simulink model "fuel_cell_vehicle"  (R2024a)
settings: Solver=VariableStepAuto  StartTime=0.0  StopTime=2474  RelTol=1e-3
libraries: autolibshared x1, slpidlib x1
settings Model: Creator=lenovo  LastModifiedBy=lenovo

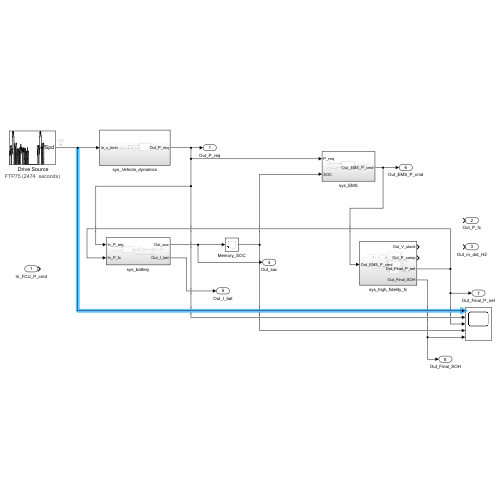
[thumbnail: Simulink's stored preview of the top-level diagram]
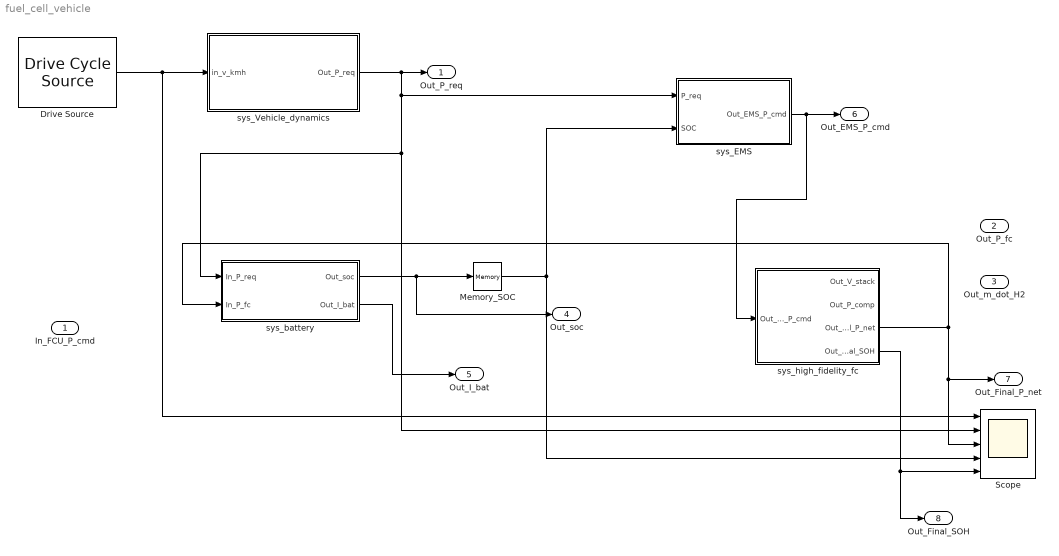
== system fuel_cell_vehicle ==
  In_FCU_P_cmd : Inport
  " Drive Source" : autolibshared/Drive Cycle Source  cycleVar=FTP75  fileVar=cycleFTP75.mat  tfinal="2474  seconds"  cycleRepeat=off  outAccPort=off  outGearPort=off  gearList=No gear data  t_wot1=5  xdot_woto=0  xdot_wot1=30  t_wot2=20  xdot_wot2=0  t_wotend=30  srcUnit=m/s  outUnit=m/s  srcAccUnit=m/s/s  outAccUnit=m/s^2  dt=0  aMode=1  faultOption=off  velBnd=2  velBndUnit=mph  inUnit=m/s  timeBnd=1  failOption=off  stopSim=off  maxFaultCnt=10  maxFaultTime=2  maxTotFaultTime=15  traceOption=off  dtTrace=1  traceWindow=10  lastDCname=FTP75  lastOutUnit=mph  lastDT=0  lastTB=1  lastSB=2  forceCalcBound=off
  Memory_SOC : Memory
  Scope : Scope  NumInputPorts=5
  sys_EMS : Subsystem
  sys_Vehicle_dynamics : Subsystem
  sys_battery : Subsystem
  sys_high_fidelity_fc : Subsystem
  Out_P_req : Outport
  Out_P_fc : Outport  Port=2
  Out_m_dot_H2 : Outport  Port=3
  Out_soc : Outport  Port=4
  Out_I_bat : Outport  Port=5
  Out_EMS_P_cmd : Outport  Port=6
  Out_Final_P_net : Outport  Port=7
  Out_Final_SOH : Outport  Port=8
  wires:
  sys_Vehicle_dynamics/1(Out_P_req) -> Scope/2, sys_battery/1(In_P_req), sys_EMS/1(P_req), Out_P_req/1
  sys_high_fidelity_fc/3(Out_Final_P_net) -> sys_battery/2(In_P_fc), Scope/3, Out_Final_P_net/1
  sys_battery/1(Out_soc) -> Memory_SOC/1, Out_soc/1
  sys_battery/2(Out_I_bat) -> Out_I_bat/1
  sys_EMS/1(Out_EMS_P_cmd) -> sys_high_fidelity_fc/1(Out_EMS_P_cmd), Out_EMS_P_cmd/1
  " Drive Source"/1 -> Scope/1, sys_Vehicle_dynamics/1(in_v_kmh)
  Memory_SOC/1 -> Scope/4, sys_EMS/2(SOC)
  sys_high_fidelity_fc/4(Out_Final_SOH) -> Out_Final_SOH/1, Scope/5

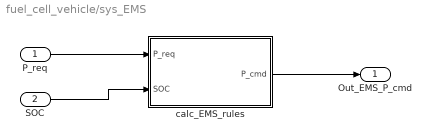
== system fuel_cell_vehicle/sys_EMS ==
  P_req : Inport
  SOC : Inport  Port=2
  calc_EMS_rules : MATLAB Function  TreatAsAtomicUnit=on
  Out_EMS_P_cmd : Outport
  wires:
  calc_EMS_rules/1(P_cmd) -> Out_EMS_P_cmd/1
  P_req/1 -> calc_EMS_rules/1(P_req)
  SOC/1 -> calc_EMS_rules/2(SOC)

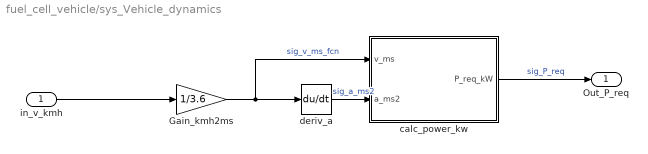
== system fuel_cell_vehicle/sys_Vehicle_dynamics ==
  in_v_kmh : Inport
  Gain_kmh2ms : Gain  Gain=1/3.6
  calc_power_kw : MATLAB Function  TreatAsAtomicUnit=on
  deriv_a : Derivative
  Out_P_req : Outport
  wires:
  in_v_kmh/1 -> Gain_kmh2ms/1
  deriv_a/1 -> calc_power_kw/2(a_ms2)  "sig_a_ms2"
  Gain_kmh2ms/1 -> deriv_a/1, calc_power_kw/1(v_ms)  "sig_v_ms_fcn"
  calc_power_kw/1(P_req_kW) -> Out_P_req/1  "sig_P_req"

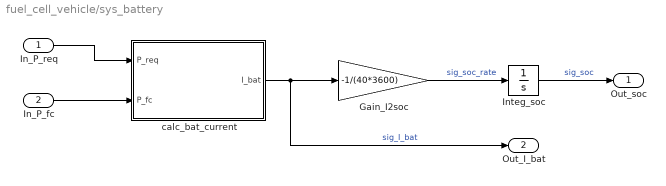
== system fuel_cell_vehicle/sys_battery ==
  In_P_req : Inport
  In_P_fc : Inport  Port=2
  Gain_I2soc : Gain  Gain=-1/(40*3600)
  Integ_soc : Integrator  InitialCondition=0.6
  calc_bat_current : MATLAB Function  TreatAsAtomicUnit=on
  Out_soc : Outport
  Out_I_bat : Outport  Port=2
  wires:
  calc_bat_current/1(I_bat) -> Out_I_bat/1, Gain_I2soc/1  "sig_I_bat"
  Gain_I2soc/1 -> Integ_soc/1  "sig_soc_rate"
  In_P_req/1 -> calc_bat_current/1(P_req)
  Integ_soc/1 -> Out_soc/1  "sig_soc"
  In_P_fc/1 -> calc_bat_current/2(P_fc)

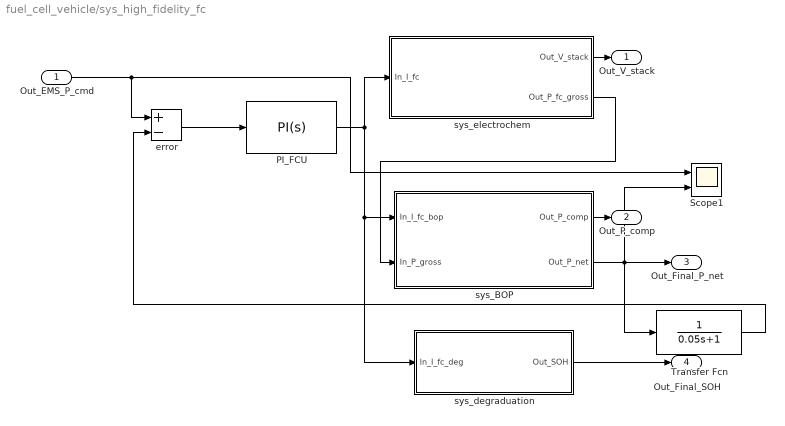
== system fuel_cell_vehicle/sys_high_fidelity_fc ==
  Out_EMS_P_cmd : Inport
  PI_FCU : slpidlib/PID Controller  Controller=PI  Form=Parallel  TimeDomain=Continuous-time  UseExternalTs=off  SampleTime=-1  IntegratorMethod=Forward Euler  FilterMethod=Forward Euler  ControllerParametersSource=internal  P=4  I=3  UseKiTs=off  D=0  UseExternalDerivativeSource=off  N=100  UseFilter=on  TunerSelectOption=Transfer Function Based (PID Tuner App)  InitialConditionSource=internal  InitialConditionForIntegrator=0  InitialConditionForFilter=0  DifferentiatorICPrevScaledInput=0  ExternalReset=none  TrackingMode=off  Kt=1  LimitOutput=on  SatLimitsSource=internal  UpperSaturationLimit=300  LowerSaturationLimit=0  LinearizeAsGain=on  AntiWindupMode=none  Kb=1  LimitIntegrator=off  UpperIntegratorSaturationLimit=inf  LowerIntegratorSaturationLimit=-inf  POutMin=[]  POutMax=[]  IOutMin=[]  IOutMax=[]  DOutMin=[]  DOutMax=[]  NOutMin=[]  NOutMax=[]  SumOutMin=[]  SumOutMax=[]  SaturationOutMin=[]  SaturationOutMax=[]  PParamMin=[]  PParamMax=[]  IParamMin=[]  IParamMax=[]  DParamMin=[]  DParamMax=[]  NParamMin=[]  NParamMax=[]  KbParamMin=[]  KbParamMax=[]  KtParamMin=[]  KtParamMax=[]  KbOutMin=[]  KbOutMax=[]  KtOutMin=[]  KtOutMax=[]  IntegratorOutMin=[]  IntegratorOutMax=[]  FilterOutMin=[]  FilterOutMax=[]  SumI1OutMin=[]  SumI1OutMax=[]  SumI2OutMin=[]  SumI2OutMax=[]  SumI3OutMin=[]  SumI3OutMax=[]  SumI4OutMin=[]  SumI4OutMax=[]  SumDOutMin=[]  SumDOutMax=[]  DifferentiatorOutMin=[]  DifferentiatorOutMax=[]  FilterDiffOutCoefMin=[]  FilterDiffOutCoefMax=[]  ReciprocalOutMin=[]  ReciprocalOutMax=[]  SumDenOutMin=[]  SumDenOutMax=[]  SumNumOutMin=[]  SumNumOutMax=[]  DivideOutMin=[]  DivideOutMax=[]  UdiffTsProdOutMin=[]  UdiffTsProdOutMax=[]  NTsProdOutMin=[]  NTsProdOutMax=[]  UintegralTsProdOutMin=[]  UintegralTsProdOutMax=[]  UngainTsProdOutMin=[]  UngainTsProdOutMax=[]  ClampingZeroOutDataTypeStr=Inherit: Inherit via back propagation  ClampingZeroOutMin=[]  ClampingZeroOutMax=[]  FilterDenConstantOutDataTypeStr=Inherit: Inherit via back propagation  FilterDenConstantOutMin=[]  FilterDenConstantOutMax=[]  PCopyOutDataTypeStr=Inherit: Inherit via back propagation  PCopyOutMin=[]  PCopyOutMax=[]  NCopyOutDataTypeStr=Inherit: Inherit via back propagation  NCopyOutMin=[]  NCopyOutMax=[]  IntegratorContinuousStateAttributes=''  IntegratorStateMustResolveToSignalObject=off  IntegratorRTWStateStorageClass=Auto  FilterContinuousStateAttributes=''  FilterStateMustResolveToSignalObject=off  FilterRTWStateStorageClass=Auto  ParallelPVariant=InternalParameters  IdealPVariant=Disabled  IVariant=InternalParameters  DVariant=Disabled  IntegratorVariant=Continuous  SatVariant=Enabled  AWVariant=Passthrough  PCopyVariant=Disabled  TRVariant=Disabled  FdbkBlocksVariant=Forward  IdealPFdbkVariant=Disabled  SatFdbkVariant=Disabled  DerivativeFilterVariant=Disabled  NVariant=Disabled  NCopyVariant=Disabled_SignalSpec  FilterICVariant=Disabled  IntegratorICVariant=InternalICs  ExternalResetVariant=Disabled  TRSumVariant=Passthrough  SumFdbkVariant=Disabled  SumVariant=Sum_PI  TsampFilterVariant=InternalTs  TsampNgainVariant=Passthrough  TsampIntegralVariant=Disabled_SignalSpec  ExternalSaturationOutDataTypeStr=Inherit: Same as second input  DerivativeSourceVariant=Disabled
  Scope1 : Scope  NumInputPorts=2
  Transfer Fcn : TransferFcn  Denominator=[0.05 1]
  error : Sum  Inputs=+-
  sys_BOP : Subsystem
  sys_degraduation : Subsystem
  sys_electrochem : Subsystem
  Out_V_stack : Outport
  Out_P_comp : Outport  Port=2
  Out_Final_P_net : Outport  Port=3
  Out_Final_SOH : Outport  Port=4
  wires:
  Out_EMS_P_cmd/1 -> Scope1/1, error/1
  PI_FCU/1 -> sys_degraduation/1(In_I_fc_deg), sys_BOP/1(In_I_fc_bop), sys_electrochem/1(In_I_fc)
  error/1 -> PI_FCU/1
  sys_BOP/2(Out_P_net) -> Out_Final_P_net/1, Transfer Fcn/1, Scope1/2
  Transfer Fcn/1 -> error/2
  sys_electrochem/1(Out_V_stack) -> Out_V_stack/1
  sys_electrochem/2(Out_P_fc_gross) -> sys_BOP/2(In_P_gross)
  sys_degraduation/1(Out_SOH) -> Out_Final_SOH/1
  sys_BOP/1(Out_P_comp) -> Out_P_comp/1

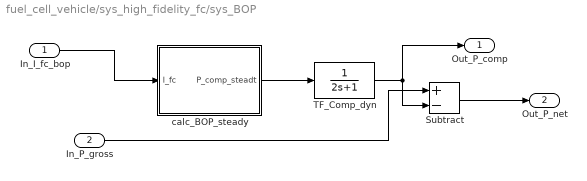
== system fuel_cell_vehicle/sys_high_fidelity_fc/sys_BOP ==
  In_I_fc_bop : Inport
  In_P_gross : Inport  Port=2
  Subtract : Sum  Inputs=+-
  TF_Comp_dyn : TransferFcn  Denominator=[2 1]
  calc_BOP_steady : MATLAB Function  TreatAsAtomicUnit=on
  Out_P_comp : Outport
  Out_P_net : Outport  Port=2
  wires:
  In_P_gross/1 -> Subtract/1
  Subtract/1 -> Out_P_net/1
  calc_BOP_steady/1(P_comp_steadt) -> TF_Comp_dyn/1
  In_I_fc_bop/1 -> calc_BOP_steady/1(I_fc)
  TF_Comp_dyn/1 -> Out_P_comp/1, Subtract/2

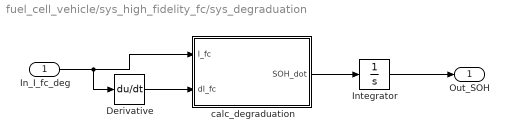
== system fuel_cell_vehicle/sys_high_fidelity_fc/sys_degraduation ==
  In_I_fc_deg : Inport
  Derivative : Derivative
  Integrator : Integrator  InitialCondition=1
  calc_degraduation : MATLAB Function  TreatAsAtomicUnit=on
  Out_SOH : Outport
  wires:
  calc_degraduation/1(SOH_dot) -> Integrator/1
  Integrator/1 -> Out_SOH/1
  In_I_fc_deg/1 -> Derivative/1, calc_degraduation/1(I_fc)
  Derivative/1 -> calc_degraduation/2(dI_fc)

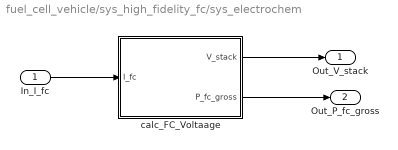
== system fuel_cell_vehicle/sys_high_fidelity_fc/sys_electrochem ==
  In_I_fc : Inport
  calc_FC_Voltaage : MATLAB Function  TreatAsAtomicUnit=on
  Out_V_stack : Outport
  Out_P_fc_gross : Outport  Port=2
  wires:
  calc_FC_Voltaage/2(P_fc_gross) -> Out_P_fc_gross/1
  In_I_fc/1 -> calc_FC_Voltaage/1(I_fc)
  calc_FC_Voltaage/1(V_stack) -> Out_V_stack/1

== matlab function fuel_cell_vehicle/sys_battery/calc_bat_current ==
  data: P_req input; I_bat output; P_fc input
function I_bat = fcn(P_req, P_fc)
    % 电池参数
    U = 300;    % 标称电压 (V)
    R = 0.1;    % 内阻 (Ohm)
    
    % 计算电池实际功率并转换为瓦特 (W)
    P_bat_W = (P_req - P_fc) * 1000;
    
    % 安全保护：防止极端大功率下根号内出现负数导致仿真崩溃
    limit_val = U^2 - 4 * R * P_bat_W;
    if limit_val < 0
        limit_val = 0; 
    end
    
    % 内阻模型计算电流 (A)
    I_bat = (U - sqrt(limit_val)) / (2 * R);
end

== matlab function fuel_cell_vehicle/sys_EMS/calc_EMS_rules ==
  data: P_req input; P_cmd output; SOC input
function P_cmd = fcn(P_req, SOC)
    % EMS 基于规则的控制策略 (Rule-based Control)
    
    % 设定阈值参数
    SOC_low = 0.4;
    SOC_high = 0.8;
    P_fc_max = 50;  % kW
    P_fc_min = 5;   % kW
    P_fc_opt = 25;  % kW
    
    % 状态机控制逻辑
    if SOC < SOC_low
        % 规则1：电量极低，强制全开充电
        P_cmd = P_fc_max;
    elseif SOC > SOC_high
        % 规则2：电量很满
        if P_req > P_fc_max
            % 如果此时车辆猛加速（需求大于FC最大功率），FC全开帮忙，保护电池
            P_cmd = P_fc_max; 
        else
            % 否则FC怠速，纯靠电池放电
            P_cmd = P_fc_min; 
        end
    else
        % 规则3：电量正常 (0.4~0.8区间)
        % 让燃料电池保持在最高效率点，剩余功率波动由电池去扛
        P_cmd = P_fc_opt; 
    end
end

== matlab function fuel_cell_vehicle/sys_high_fidelity_fc/sys_BOP/calc_BOP_steady ==
  data: I_fc input; P_comp_steadt output
function P_comp_steadt = fcn(I_fc)
c0 =0.4;
c1 =0.008;
c2=0.00007;

P_comp_steadt = c0+c1*I_fc+c2*(I_fc^2);

== matlab function fuel_cell_vehicle/sys_high_fidelity_fc/sys_degraduation/calc_degraduation ==
  data: I_fc input; SOH_dot output; dI_fc input
function SOH_dot = fcn(I_fc, dI_fc)
    % 仿真加速因子（放大 10000 倍，以便在短时间仿真中能肉眼看到寿命下降）
    Acc_Factor = 100;
    
    % 寿命衰减参数
    I_opt = 100;         % 最佳健康电流 (A)
    k0 = 5e-7;           % 基础衰减率
    k1 = 2e-11;          % 稳态偏离惩罚系数
    k_trans = 1e-6;      % 动态突变惩罚系数
    
    % 计算稳态衰减 (偏离 100A 越远，衰减越快)
    k_steady = k0 + k1 * (I_fc - I_opt)^2;
    
    % 计算瞬态突变衰减 (电流变化越剧烈，衰减越快)
    k_dynamic = k_trans * abs(dI_fc);
    
    % 总衰减率 (D_dot 为正，表示每秒扣除的健康度)
    D_dot = (k_steady + k_dynamic) * Acc_Factor;
    
    % 健康度变化率 (输出负值，方便直接积分)
    SOH_dot = -D_dot;
end

== matlab function fuel_cell_vehicle/sys_high_fidelity_fc/sys_electrochem/calc_FC_Voltaage ==
  data: I_fc input; V_stack output; P_fc_gross output
function [V_stack, P_fc_gross] = fcn(I_fc)
    % 燃料电池电化学半经验参数 (60kW 级标定)
    N = 300;        % 串联电池片数
    E0 = 1.1;       % 开路电压 (V)
    A = 0.03;       % 激活极化常数 (V)
    R_ohm = 0.0002; % 欧姆极化内阻 (Ohm)
    B = 0.05;       % 浓差极化常数 (V)
    I_max = 300;    % 极限电流 (A)
    
    % 安全限幅：防止电流超限导致 ln(负数) 报错崩溃
    if I_fc >= I_max - 1
        I_fc = I_max - 1;
    elseif I_fc < 0
        I_fc = 0;
    end
    
    % 计算三大极化电压降
    V_act = A * log(I_fc + 1);                       % 激活极化
    V_ohm = R_ohm * I_fc;                            % 欧姆极化
    V_conc = -B * log(1 - (I_fc / I_max));           % 浓差极化
    
    % 单片电池真实电压
    V_cell = E0 - V_act - V_ohm - V_conc;
    
    % 安全限幅：防止电压变成负数
    if V_cell < 0
        V_cell = 0;
    end
    
    % 计算电堆总电压与总功率 (kW)
    V_stack = N * V_cell;
    P_fc_gross = (V_stack * I_fc) / 1000;
end

== matlab function fuel_cell_vehicle/sys_Vehicle_dynamics/calc_power_kw ==
  data: v_ms input; P_req_kW output; a_ms2 input
function P_req_kW = fcn(v_ms, a_ms2)
    % 车辆固定参数
    m = 1500;   % 质量
    g = 9.81;   % 重力加速度
    Cr = 0.01;  % 滚阻系数
    rho = 1.2;  % 空气密度
    Cd = 0.3;   % 风阻系数
    A = 2.2;    % 迎风面积
    
    % 计算三大阻力 (单位: N)
    F_roll = m * g * Cr;                            % 滚动阻力
    F_air = 0.5 * rho * Cd * A * (v_ms^2);          % 空气阻力
    F_acc = m * a_ms2;                              % 加速阻力
    
    % 计算总阻力并转化为千瓦功率 (kW)
    F_total = F_roll + F_air + F_acc;
    P_req_kW = (F_total * v_ms) / 1000;
end
